simulink model "InvDyn_PID_Point_Point"  (R2022b)
settings: Solver=VariableStepAuto  StartTime=0.0  StopTime=10.0  RelTol=1e-3
settings Model: Creator=AD  LastModifiedBy=AD

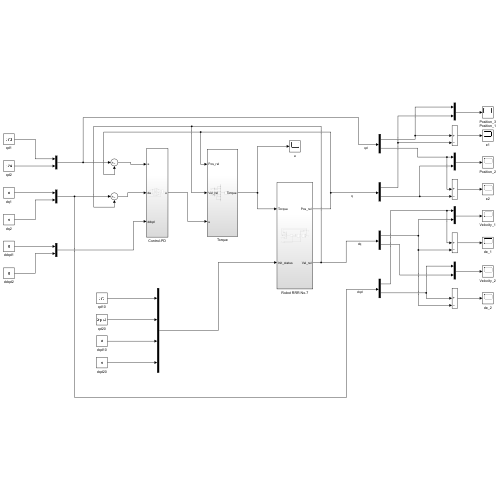
[thumbnail: Simulink's stored preview of the top-level diagram]
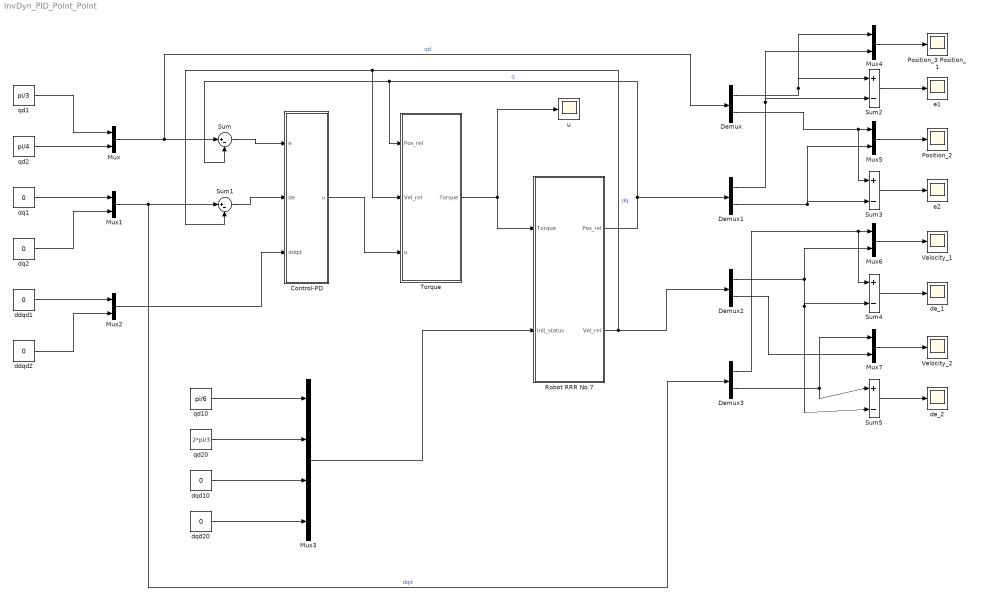
== system InvDyn_PID_Point_Point ==
  Control-PD : Subsystem
  Demux{,1..3} (4 alike) : Demux  Outputs=2
  Mux{,1..2,4..7} (7 alike) : Mux  Inputs=2
  Mux3 : Mux
  Position_2 : Scope
  Position_3 Position_1 : Scope
  Robot RRR No.7 : Subsystem
  Sum{,1..5} (6 alike) : Sum  Inputs=|+-
  Torque : Subsystem
  Velocity_1 : Scope
  Velocity_2 : Scope
  ddqd1 : Constant  Value=0
  ddqd2 : Constant  Value=0
  de_1 : Scope
  de_2 : Scope
  dq1 : Constant  Value=0
  dq2 : Constant  Value=0
  dqd10 : Constant  Value=0
  dqd20 : Constant  Value=0
  e1 : Scope
  e2 : Scope
  qd1 : Constant  Value=pi/3
  qd10 : Constant  Value=pi/6
  qd2 : Constant  Value=pi/4
  qd20 : Constant  Value=2*pi/3
  u : Scope
  wires:
  qd1/1 -> Mux/1
  qd2/1 -> Mux/2
  dq1/1 -> Mux1/1
  dq2/1 -> Mux1/2
  ddqd1/1 -> Mux2/1
  ddqd2/1 -> Mux2/2
  Mux/1 -> Demux/1, Sum/1  "qd"
  Mux1/1 -> Sum1/1, Demux3/1  "dqd"
  Sum1/1 -> Control-PD/2(de)
  Sum/1 -> Control-PD/1(e)
  Mux2/1 -> Control-PD/3(ddqd)
  qd20/1 -> Mux3/2
  qd10/1 -> Mux3/1
  dqd10/1 -> Mux3/3
  dqd20/1 -> Mux3/4
  Torque/1(Torque) -> Robot RRR No.7/1(Torque), u/1
  Mux3/1 -> Robot RRR No.7/2(Init_status)
  Sum4/1 -> de_1/1
  Mux6/1 -> Velocity_1/1
  Sum3/1 -> e2/1
  Mux5/1 -> Position_2/1
  Mux4/1 -> Position_3 Position_1/1
  Sum2/1 -> e1/1
  Mux7/1 -> Velocity_2/1
  Sum5/1 -> de_2/1
  Demux/1 -> Sum2/1, Mux4/1
  Demux/2 -> Sum3/1, Mux5/1
  Demux1/1 -> Sum2/2, Mux4/2
  Demux1/2 -> Sum3/2, Mux5/2
  Demux2/1 -> Mux6/2, Sum4/2, Sum5/2
  Demux2/2 -> Mux7/2
  Demux3/1 -> Sum4/1, Mux6/1
  Demux3/2 -> Sum5/1, Mux7/1
  Robot RRR No.7/1(Pos_rel) -> Torque/1(Pos_rel), Sum/2, Demux1/1  "q"
  Robot RRR No.7/2(Vel_rel) -> Torque/2(Vel_rel), Sum1/2, Demux2/1  "dq"
  Control-PD/1(u) -> Torque/3(u)

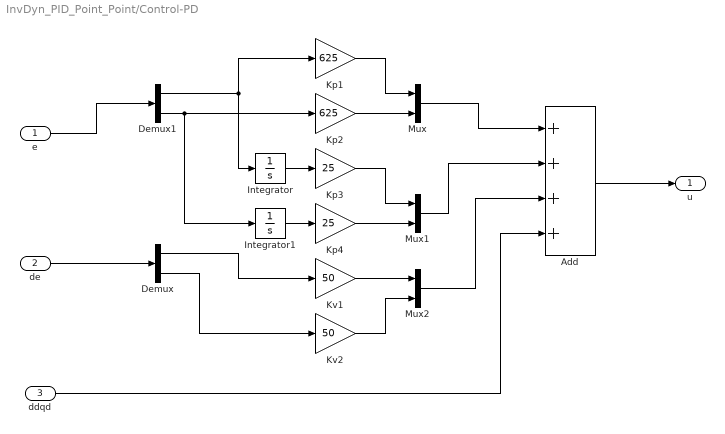
== system InvDyn_PID_Point_Point/Control-PD ==
  e : Inport
  de : Inport  Port=2
  ddqd : Inport  Port=3
  Add : Sum  Inputs=++++
  Demux : Demux  Outputs=2
  Demux1 : Demux  Outputs=2
  Integrator : Integrator
  Integrator1 : Integrator
  Kp1 : Gain  Gain=625
  Kp2 : Gain  Gain=625
  Kp3 : Gain  Gain=25
  Kp4 : Gain  Gain=25
  Kv1 : Gain  Gain=50
  Kv2 : Gain  Gain=50
  Mux : Mux  Inputs=2
  Mux1 : Mux  Inputs=2
  Mux2 : Mux  Inputs=2
  u : Outport
  wires:
  e/1 -> Demux1/1
  de/1 -> Demux/1
  Demux1/1 -> Integrator/1, Kp1/1
  Integrator/1 -> Kp3/1
  Demux1/2 -> Integrator1/1, Kp2/1
  Integrator1/1 -> Kp4/1
  Demux/1 -> Kv1/1
  Demux/2 -> Kv2/1
  Kp1/1 -> Mux/1
  Kp2/1 -> Mux/2
  Kp3/1 -> Mux1/1
  Kp4/1 -> Mux1/2
  Kv1/1 -> Mux2/1
  Kv2/1 -> Mux2/2
  ddqd/1 -> Add/4
  Mux2/1 -> Add/3
  Mux1/1 -> Add/2
  Mux/1 -> Add/1
  Add/1 -> u/1

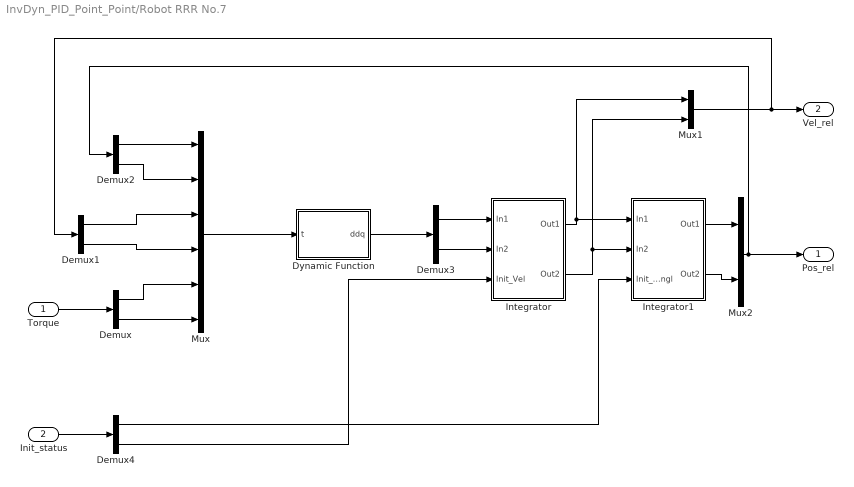
== system InvDyn_PID_Point_Point/Robot RRR No.7 ==
  Torque : Inport
  Init_status : Inport  Port=2
  Demux{,1..4} (5 alike) : Demux  Outputs=2
  Dynamic Function : MATLAB Function  TreatAsAtomicUnit=on
  Integrator : Subsystem
  Integrator1 : Subsystem
  Mux : Mux  Inputs=6
  Mux1 : Mux  Inputs=2
  Mux2 : Mux  Inputs=2
  Pos_rel : Outport
  Vel_rel : Outport  Port=2
  wires:
  Demux2/1 -> Mux/1
  Demux2/2 -> Mux/2
  Demux1/1 -> Mux/3
  Demux1/2 -> Mux/4
  Demux/1 -> Mux/5
  Demux/2 -> Mux/6
  Dynamic Function/1(ddq) -> Demux3/1
  Demux3/1 -> Integrator/1(In1)
  Demux3/2 -> Integrator/2(In2)
  Mux/1 -> Dynamic Function/1(t)
  Torque/1 -> Demux/1
  Init_status/1 -> Demux4/1
  Demux4/2 -> Integrator/3(Init_Vel)
  Demux4/1 -> Integrator1/3(Init_Angl)
  Integrator/1(Out1) -> Mux1/1, Integrator1/1(In1)
  Integrator/2(Out2) -> Mux1/2, Integrator1/2(In2)
  Integrator1/1(Out1) -> Mux2/1
  Integrator1/2(Out2) -> Mux2/2
  Mux2/1 -> Demux2/1, Pos_rel/1
  Mux1/1 -> Demux1/1, Vel_rel/1

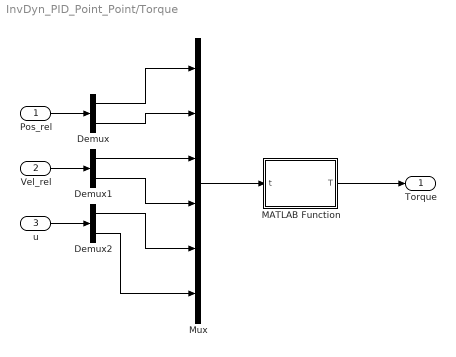
== system InvDyn_PID_Point_Point/Torque ==
  Pos_rel : Inport
  Vel_rel : Inport  Port=2
  u : Inport  Port=3
  Demux : Demux  Outputs=2
  Demux1 : Demux  Outputs=2
  Demux2 : Demux  Outputs=2
  MATLAB Function : MATLAB Function  TreatAsAtomicUnit=on
  Mux : Mux  Inputs=6
  Torque : Outport
  wires:
  Pos_rel/1 -> Demux/1
  Demux/1 -> Mux/1
  Demux/2 -> Mux/2
  Demux1/1 -> Mux/3
  Vel_rel/1 -> Demux1/1
  Demux1/2 -> Mux/4
  u/1 -> Demux2/1
  Demux2/1 -> Mux/5
  Demux2/2 -> Mux/6
  Mux/1 -> MATLAB Function/1(t)
  MATLAB Function/1(T) -> Torque/1

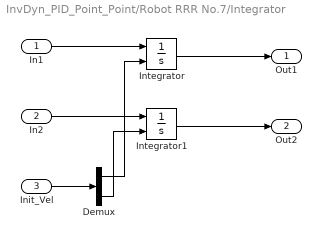
== system InvDyn_PID_Point_Point/Robot RRR No.7/Integrator ==
  In1 : Inport
  In2 : Inport  Port=2
  Init_Vel : Inport  Port=3
  Demux : Demux  Outputs=2
  Integrator : Integrator  InitialConditionSource=external
  Integrator1 : Integrator  InitialConditionSource=external
  Out1 : Outport
  Out2 : Outport  Port=2
  wires:
  In1/1 -> Integrator/1
  Init_Vel/1 -> Demux/1
  Demux/1 -> Integrator/2
  Demux/2 -> Integrator1/2
  In2/1 -> Integrator1/1
  Integrator/1 -> Out1/1
  Integrator1/1 -> Out2/1

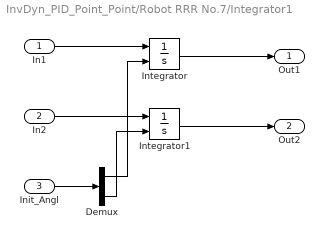
== system InvDyn_PID_Point_Point/Robot RRR No.7/Integrator1 ==
  In1 : Inport
  In2 : Inport  Port=2
  Init_Angl : Inport  Port=3
  Demux : Demux  Outputs=2
  Integrator : Integrator  InitialConditionSource=external
  Integrator1 : Integrator  InitialConditionSource=external
  Out1 : Outport
  Out2 : Outport  Port=2
  wires:
  In1/1 -> Integrator/1
  Init_Angl/1 -> Demux/1
  Demux/1 -> Integrator/2
  Demux/2 -> Integrator1/2
  In2/1 -> Integrator1/1
  Integrator/1 -> Out1/1
  Integrator1/1 -> Out2/1

== matlab function InvDyn_PID_Point_Point/Torque/MATLAB Function ==
  data: t input; T output
function T = InverseModel(t)
m1 = 15; m2 = 8;
a1 = 0.33; a2 = 0.33;
g = 9.81;

Fx = 20; Fy = 20; Mz = 10;

q = t(1:2);
dq = t(3:4);
u = t(5:6);

m11 = (m1/3+m2)*a1^2 + (m2/3)*a2^2 + m2*a1*a2*cos(q(2));
m12 = (m2/2)*a1*a2*cos(q(2)) + (m2/3)*a2^2;
m21 = m12;
m22 = m2*a2^2/3;

M = [m11,m12;m21,m22];

psi1 = -m2*a1*a2*sin(q(2)) - m2*a1*a2*sin(q(2))/2;
psi2 = m2*a1*a2*sin(q(2))*dq(1)^2/2;

Psi = [psi1;psi2];

g1 = (m1/2+m2)*g*a1*cos(q(1))+m2*g/2*a2*cos(q(1)+q(2));
g2 = m2*g/2*a2*cos(q(1)+q(2));

G = [g1; g2];

Q1=-(a1*sin(q(1))+a2*sin(q(1)+q(2)))*Fx+(a1*cos(q(1))+a2*cos(q(1)+q(2)))*Fy+Mz;
Q2=-a2*sin(q(1)+q(2))*Fx+a2*cos(q(1)+q(2))*Fy+Mz;

Q = [Q1;Q2];

T = M*[u(1);u(2)]+Psi+G+Q;

== matlab function InvDyn_PID_Point_Point/Robot RRR No.7/Dynamic Function ==
  data: t input; ddq output
function ddq = RobotDynamics(t)

m1 = 15; m2 = 8;
a1 = 0.33; a2 = 0.33;
g = 9.81;

Fx = 20; Fy = 20; Mz = 10;

q = t(1:2);
dq = t(3:4);
U = t(5:6);

% Ma tran khoi luong
m11=(m1/3+m2)*a1^2+(m2/3)*a2^2+m2*a1*a2*cos(q(2)); 
m12 = (m2/2)*a1*a2*cos(q(2))+(m2/3)*a2^2;

m21 = m12;
m22 = m2*a2^2/3;

M = [m11,m12;m21,m22];

% Luc qun tinh coriolis  va qun tinh li tam
psi1 = -m2*a1*a2*sin(q(2))-m2*a1*a2*sin(q(2))/2;
psi2 = m2*a1*a2*sin(q(2))*dq(1)^2/2;

Psi=[psi1;psi2];

% Luc suy rong cua cac luc co the
g1 = (m1/2+m2)*g*a1*cos(q(1))+m2*g/2*a2*cos(q(1)+q(2));
g2 = m2*g/2*a2*cos(q(1)+q(2));

G = [g1; g2];

% Luc suy rong cua cac luc khong the
%Q1=0.2*dq(1);
%Q2=0.2*dq(2);

Q1=-(a1*sin(q(1))+a2*sin(q(1)+q(2)))*Fx+(a1*cos(q(1))+a2*cos(q(1)+q(2)))*Fy+Mz;
Q2=-a2*sin(q(1)+q(2))*Fx+a2*cos(q(1)+q(2))*Fy+Mz;

Q=[Q1;Q2];

ddq = inv(M)*([U(1);U(2)]-Psi-G-Q);
